simulink model "pompa"  (R2022b)
settings: Solver=VariableStepAuto  StartTime=0.0  StopTime=10.0  RelTol=1e-3
values from neighbouring files (symbols this model uses):
  k11 = k2^2+4*(k-k3)*k1    (= 0.1090506)    [run_first.m]
  k12 = 8*(k-k3)    (= 0.3488)    [run_first.m]
  k13 = 2*(k-k3)    (= 0.0872)    [run_first.m]
  k2 = -0.015    [run_first.m]
settings Model: Creator=fabian  LastModifiedBy=fabian
settings ModelReferenceCC: ModelReferenceMinAlgLoopOccurrences=on

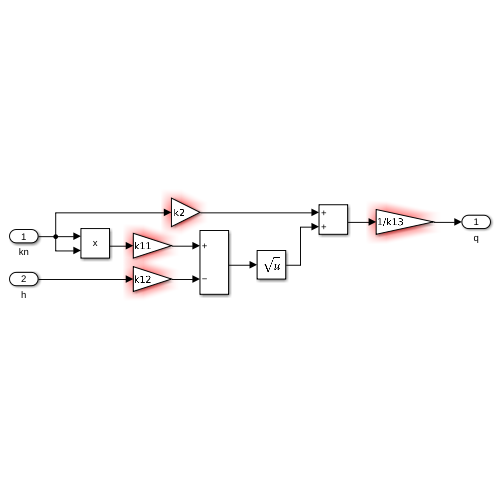
[thumbnail: Simulink's stored preview of the top-level diagram]
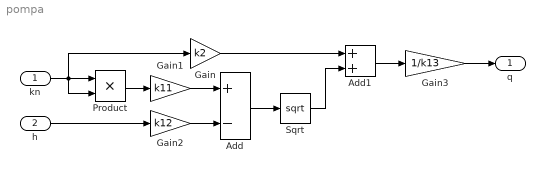
== system pompa ==
  kn : Inport
  h : Inport  Port=2
  Add : Sum  Inputs=+-
  Add1 : Sum
  Gain : Gain  Gain=k2
  Gain1 : Gain  Gain=k11
  Gain2 : Gain  Gain=k12
  Gain3 : Gain  Gain=1/k13
  Product : Product
  Sqrt : Sqrt
  q : Outport
  wires:
  kn/1 -> Gain/1, Product/1, Product/2
  Product/1 -> Gain1/1
  h/1 -> Gain2/1
  Gain1/1 -> Add/1
  Gain2/1 -> Add/2
  Add/1 -> Sqrt/1
  Gain/1 -> Add1/1
  Sqrt/1 -> Add1/2
  Add1/1 -> Gain3/1
  Gain3/1 -> q/1
